simulink model "stateflow_calculator"  (R2017b)
settings: Solver=FixedStepDiscrete  StartTime=0.0  StopTime=10.0  RelTol=1e-3
settings Model: Creator=ibrahim  LastModifiedBy=ibrahim
settings OptimizationCC: DefaultParameterBehavior=Inlined  PassReuseOutputArgsAs=Individual arguments
settings DebuggingCC: ParameterTunabilityLossMsg=error
settings SFSimCC: MATLABDynamicMemAlloc=off
settings RTWCC: SystemTargetFile=ert.tlc  GenCodeOnly=on  TemplateMakefile=ert_default_tmf  GenerateReport=on  IncludeHyperlinkInReport=on  LaunchReport=on  GenerateTraceInfo=on  GenerateTraceReport=on  GenerateTraceReportSl=on  GenerateTraceReportSf=on  GenerateTraceReportEml=on  GenerateWebview=on
settings CodeAppCC: ForceParamTrailComments=on  IgnoreCustomStorageClasses=off  OperatorAnnotations=on  SimulinkDataObjDesc=on  SFDataObjDesc=on  InsertBlockDesc=on
settings ERTTargetCC: TargetLangStandard=C99 (ISO)  GenerateSampleERTMain=on  InlinedParameterPlacement=NonHierarchical  ERTCustomFileTemplate=example_file_process.tlc

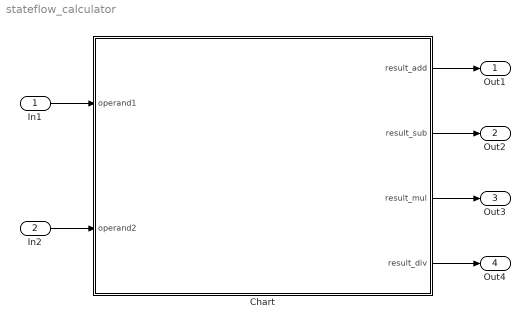
== system stateflow_calculator ==
  In1 : Inport
  In2 : Inport  Port=2
  Chart : Stateflow chart  TreatAsAtomicUnit=on
  Out1 : Outport
  Out2 : Outport  Port=2
  Out3 : Outport  Port=3
  Out4 : Outport  Port=4
  wires:
  In1/1 -> Chart/1(operand1)
  In2/1 -> Chart/2(operand2)
  Chart/1(result_add) -> Out1/1
  Chart/2(result_sub) -> Out2/1
  Chart/3(result_mul) -> Out3/1
  Chart/4(result_div) -> Out4/1

== stateflow chart stateflow_calculator/Chart ==
  (default) -> (junction 7)
  (junction 7) -> (junction 14) : {result_add = operand1 + operand2;
      | 		result_sub = operand1 - operand2;
      | 		result_mul = operand1 * operand2;}
  (junction 14) -> (junction 24)
  (junction 24) -> (junction 25) [order 1] : [operand2 != 0]
  (junction 24) -> (junction 26) [order 2]
  (junction 25) -> (junction 27) : {result_div = operand1 / operand2;}
  (junction 27) -> (junction 26)
  (junction 26) -> (junction 28)
  data: operand1 input; operand2 input; result_add output; result_sub output double; result_mul output double; result_div output double
